simulink model "NeuralcircuitULInjured08102023_DSD"  (R2023a)
settings: Solver=VariableStepAuto  StartTime=0.0  StopTime=1600  RelTol=1e-3
values from neighbouring files (symbols this model uses):
  Cn = 1    [Inhibitory_excitatory_ULInjury_1Hz_08102023.m]    (also in Inhibitory_excitatory_ULInjury_30Hz_08102023.m; InitialExcitatoryInhibitoryNeurons_Healthy08062023.m; InitialExcitatoryInhibitoryULInjured_08102023_DSD.m)
  EK = -84*1    (= -84)    [Inhibitory_excitatory_ULInjury_1Hz_08102023.m]    (also in Inhibitory_excitatory_ULInjury_30Hz_08102023.m; InitialExcitatoryInhibitoryNeurons_Healthy08062023.m; InitialExcitatoryInhibitoryULInjured_08102023_DSD.m)
  EKEx = -90    [Inhibitory_excitatory_ULInjury_1Hz_08102023.m]    (also in Inhibitory_excitatory_ULInjury_30Hz_08102023.m; InitialExcitatoryInhibitoryNeurons_Healthy08062023.m; InitialExcitatoryInhibitoryULInjured_08102023_DSD.m)
  EKIn = -90    [Inhibitory_excitatory_ULInjury_1Hz_08102023.m]    (also in Inhibitory_excitatory_ULInjury_30Hz_08102023.m; InitialExcitatoryInhibitoryNeurons_Healthy08062023.m; InitialExcitatoryInhibitoryULInjured_08102023_DSD.m)
  ELEx = -65    [Inhibitory_excitatory_ULInjury_1Hz_08102023.m]    (also in Inhibitory_excitatory_ULInjury_30Hz_08102023.m; InitialExcitatoryInhibitoryNeurons_Healthy08062023.m; InitialExcitatoryInhibitoryULInjured_08102023_DSD.m)
  ELIn = -65    [Inhibitory_excitatory_ULInjury_1Hz_08102023.m]    (also in Inhibitory_excitatory_ULInjury_30Hz_08102023.m; InitialExcitatoryInhibitoryNeurons_Healthy08062023.m; InitialExcitatoryInhibitoryULInjured_08102023_DSD.m)
  ELk = -83.38*1    (= -83.38)    [Inhibitory_excitatory_ULInjury_1Hz_08102023.m]    (also in Inhibitory_excitatory_ULInjury_30Hz_08102023.m; InitialExcitatoryInhibitoryNeurons_Healthy08062023.m; InitialExcitatoryInhibitoryULInjured_08102023_DSD.m)
  ENa = 50*1    (= 50)    [Inhibitory_excitatory_ULInjury_1Hz_08102023.m]    (also in Inhibitory_excitatory_ULInjury_30Hz_08102023.m; InitialExcitatoryInhibitoryNeurons_Healthy08062023.m; InitialExcitatoryInhibitoryULInjured_08102023_DSD.m)
  ENaEx = 60    [Inhibitory_excitatory_ULInjury_1Hz_08102023.m]    (also in Inhibitory_excitatory_ULInjury_30Hz_08102023.m; InitialExcitatoryInhibitoryNeurons_Healthy08062023.m; InitialExcitatoryInhibitoryULInjured_08102023_DSD.m)
  ENaIn = 55    [Inhibitory_excitatory_ULInjury_1Hz_08102023.m]    (also in Inhibitory_excitatory_ULInjury_30Hz_08102023.m; InitialExcitatoryInhibitoryNeurons_Healthy08062023.m; InitialExcitatoryInhibitoryULInjured_08102023_DSD.m)
  ErestE = -65    [Inhibitory_excitatory_ULInjury_1Hz_08102023.m]    (also in Inhibitory_excitatory_ULInjury_30Hz_08102023.m; InitialExcitatoryInhibitoryNeurons_Healthy08062023.m; InitialExcitatoryInhibitoryULInjured_08102023_DSD.m)
  ErestIn = -64    [Inhibitory_excitatory_ULInjury_1Hz_08102023.m]    (also in Inhibitory_excitatory_ULInjury_30Hz_08102023.m; InitialExcitatoryInhibitoryNeurons_Healthy08062023.m; InitialExcitatoryInhibitoryULInjured_08102023_DSD.m)
  ESynE = -10    [Inhibitory_excitatory_ULInjury_1Hz_08102023.m]    (also in Inhibitory_excitatory_ULInjury_30Hz_08102023.m; InitialExcitatoryInhibitoryNeurons_Healthy08062023.m; InitialExcitatoryInhibitoryULInjured_08102023_DSD.m)
  ESynE2 = -10    [Inhibitory_excitatory_ULInjury_1Hz_08102023.m]    (also in Inhibitory_excitatory_ULInjury_30Hz_08102023.m; InitialExcitatoryInhibitoryNeurons_Healthy08062023.m; InitialExcitatoryInhibitoryULInjured_08102023_DSD.m)
  ESynE3 = -10    [Inhibitory_excitatory_ULInjury_1Hz_08102023.m]    (also in Inhibitory_excitatory_ULInjury_30Hz_08102023.m; InitialExcitatoryInhibitoryNeurons_Healthy08062023.m; InitialExcitatoryInhibitoryULInjured_08102023_DSD.m)
  ESynE4 = -10    [Inhibitory_excitatory_ULInjury_1Hz_08102023.m]    (also in Inhibitory_excitatory_ULInjury_30Hz_08102023.m; InitialExcitatoryInhibitoryNeurons_Healthy08062023.m; InitialExcitatoryInhibitoryULInjured_08102023_DSD.m)
  ESynE5 = -10    [Inhibitory_excitatory_ULInjury_1Hz_08102023.m]    (also in Inhibitory_excitatory_ULInjury_30Hz_08102023.m; InitialExcitatoryInhibitoryNeurons_Healthy08062023.m; InitialExcitatoryInhibitoryULInjured_08102023_DSD.m)
  ESynE6 = -15    [Inhibitory_excitatory_ULInjury_1Hz_08102023.m]    (also in Inhibitory_excitatory_ULInjury_30Hz_08102023.m; InitialExcitatoryInhibitoryNeurons_Healthy08062023.m; InitialExcitatoryInhibitoryULInjured_08102023_DSD.m = -10)
  ESynE7 = -10    [Inhibitory_excitatory_ULInjury_1Hz_08102023.m]    (also in Inhibitory_excitatory_ULInjury_30Hz_08102023.m; InitialExcitatoryInhibitoryNeurons_Healthy08062023.m; InitialExcitatoryInhibitoryULInjured_08102023_DSD.m)
  ESynI = -80    [Inhibitory_excitatory_ULInjury_1Hz_08102023.m]    (also in Inhibitory_excitatory_ULInjury_30Hz_08102023.m; InitialExcitatoryInhibitoryNeurons_Healthy08062023.m; InitialExcitatoryInhibitoryULInjured_08102023_DSD.m)
  ESynI2 = -80    [Inhibitory_excitatory_ULInjury_1Hz_08102023.m]    (also in Inhibitory_excitatory_ULInjury_30Hz_08102023.m; InitialExcitatoryInhibitoryNeurons_Healthy08062023.m; InitialExcitatoryInhibitoryULInjured_08102023_DSD.m)
  ESynI3 = -80    [Inhibitory_excitatory_ULInjury_1Hz_08102023.m]    (also in Inhibitory_excitatory_ULInjury_30Hz_08102023.m; InitialExcitatoryInhibitoryNeurons_Healthy08062023.m; InitialExcitatoryInhibitoryULInjured_08102023_DSD.m)
  ESynI5 = -80    [Inhibitory_excitatory_ULInjury_1Hz_08102023.m]    (also in Inhibitory_excitatory_ULInjury_30Hz_08102023.m; InitialExcitatoryInhibitoryNeurons_Healthy08062023.m; InitialExcitatoryInhibitoryULInjured_08102023_DSD.m)
  ESynI6 = -65    [Inhibitory_excitatory_ULInjury_1Hz_08102023.m]    (also in Inhibitory_excitatory_ULInjury_30Hz_08102023.m; InitialExcitatoryInhibitoryNeurons_Healthy08062023.m; InitialExcitatoryInhibitoryULInjured_08102023_DSD.m = -80)
  Exh0 = ahEx(V0)./(ahEx(V0)+bhEx(V0))    [Inhibitory_excitatory_ULInjury_1Hz_08102023.m]    (also in Inhibitory_excitatory_ULInjury_30Hz_08102023.m; InitialExcitatoryInhibitoryNeurons_Healthy08062023.m; InitialExcitatoryInhibitoryULInjured_08102023_DSD.m)
  Exm0 = amEx(V0)./(amEx(V0)+bmEx(V0))    [Inhibitory_excitatory_ULInjury_1Hz_08102023.m]    (also in Inhibitory_excitatory_ULInjury_30Hz_08102023.m; InitialExcitatoryInhibitoryNeurons_Healthy08062023.m; InitialExcitatoryInhibitoryULInjured_08102023_DSD.m)
  Exn0 = anEx(V0)./(anEx(V0)+bnEx(V0))    [Inhibitory_excitatory_ULInjury_1Hz_08102023.m]    (also in Inhibitory_excitatory_ULInjury_30Hz_08102023.m; InitialExcitatoryInhibitoryNeurons_Healthy08062023.m; InitialExcitatoryInhibitoryULInjured_08102023_DSD.m)
  Ga = 1*Gaxial    (= 0.351233961271)    [Inhibitory_excitatory_ULInjury_1Hz_08102023.m]    (also in Inhibitory_excitatory_ULInjury_30Hz_08102023.m; InitialExcitatoryInhibitoryNeurons_Healthy08062023.m; InitialExcitatoryInhibitoryULInjured_08102023_DSD.m)
  Gaxial = pi*(d^2)/(4*Ro_ax*Internodal_L)*1e7    (= 0.351233961271)    [Inhibitory_excitatory_ULInjury_1Hz_08102023.m]    (also in Inhibitory_excitatory_ULInjury_30Hz_08102023.m; InitialExcitatoryInhibitoryNeurons_Healthy08062023.m; InitialExcitatoryInhibitoryULInjured_08102023_DSD.m)
  gKEx = 100    [Inhibitory_excitatory_ULInjury_1Hz_08102023.m]    (also in Inhibitory_excitatory_ULInjury_30Hz_08102023.m; InitialExcitatoryInhibitoryNeurons_Healthy08062023.m; InitialExcitatoryInhibitoryULInjured_08102023_DSD.m)
  gKIn = 9    [Inhibitory_excitatory_ULInjury_1Hz_08102023.m]    (also in Inhibitory_excitatory_ULInjury_30Hz_08102023.m; InitialExcitatoryInhibitoryNeurons_Healthy08062023.m; InitialExcitatoryInhibitoryULInjured_08102023_DSD.m)
  gKs = 10*0.08/1    (= 0.8)    [Inhibitory_excitatory_ULInjury_1Hz_08102023.m]    (also in Inhibitory_excitatory_ULInjury_30Hz_08102023.m; InitialExcitatoryInhibitoryNeurons_Healthy08062023.m; InitialExcitatoryInhibitoryULInjured_08102023_DSD.m)
  gLEx = 0.1    [Inhibitory_excitatory_ULInjury_1Hz_08102023.m]    (also in Inhibitory_excitatory_ULInjury_30Hz_08102023.m; InitialExcitatoryInhibitoryNeurons_Healthy08062023.m; InitialExcitatoryInhibitoryULInjured_08102023_DSD.m)
  gLIn = 0.1    [Inhibitory_excitatory_ULInjury_1Hz_08102023.m]    (also in Inhibitory_excitatory_ULInjury_30Hz_08102023.m; InitialExcitatoryInhibitoryNeurons_Healthy08062023.m; InitialExcitatoryInhibitoryULInjured_08102023_DSD.m)
  gLk = 10*0.08/1    (= 0.8)    [Inhibitory_excitatory_ULInjury_1Hz_08102023.m]    (also in Inhibitory_excitatory_ULInjury_30Hz_08102023.m; InitialExcitatoryInhibitoryNeurons_Healthy08062023.m; InitialExcitatoryInhibitoryULInjured_08102023_DSD.m)
  gNaEx = 30    [Inhibitory_excitatory_ULInjury_1Hz_08102023.m]    (also in Inhibitory_excitatory_ULInjury_30Hz_08102023.m; InitialExcitatoryInhibitoryNeurons_Healthy08062023.m; InitialExcitatoryInhibitoryULInjured_08102023_DSD.m)
  gNaf = 10*3/1    (= 30)    [Inhibitory_excitatory_ULInjury_1Hz_08102023.m]    (also in Inhibitory_excitatory_ULInjury_30Hz_08102023.m; InitialExcitatoryInhibitoryNeurons_Healthy08062023.m; InitialExcitatoryInhibitoryULInjured_08102023_DSD.m)
  gNaIn = 35    [Inhibitory_excitatory_ULInjury_1Hz_08102023.m]    (also in Inhibitory_excitatory_ULInjury_30Hz_08102023.m; InitialExcitatoryInhibitoryNeurons_Healthy08062023.m; InitialExcitatoryInhibitoryULInjured_08102023_DSD.m)
  gNap = 10*0.005/1    (= 0.05)    [Inhibitory_excitatory_ULInjury_1Hz_08102023.m]    (also in Inhibitory_excitatory_ULInjury_30Hz_08102023.m; InitialExcitatoryInhibitoryNeurons_Healthy08062023.m; InitialExcitatoryInhibitoryULInjured_08102023_DSD.m)
  gSynE = 0.08    [Inhibitory_excitatory_ULInjury_1Hz_08102023.m]    (also in Inhibitory_excitatory_ULInjury_30Hz_08102023.m; InitialExcitatoryInhibitoryNeurons_Healthy08062023.m; InitialExcitatoryInhibitoryULInjured_08102023_DSD.m)
  gSynE2 = 0.08    [Inhibitory_excitatory_ULInjury_1Hz_08102023.m]    (also in Inhibitory_excitatory_ULInjury_30Hz_08102023.m; InitialExcitatoryInhibitoryNeurons_Healthy08062023.m; InitialExcitatoryInhibitoryULInjured_08102023_DSD.m)
  gSynE3 = 0.08    [Inhibitory_excitatory_ULInjury_1Hz_08102023.m]    (also in Inhibitory_excitatory_ULInjury_30Hz_08102023.m; InitialExcitatoryInhibitoryNeurons_Healthy08062023.m; InitialExcitatoryInhibitoryULInjured_08102023_DSD.m)
  gSynE4 = 0.08    [Inhibitory_excitatory_ULInjury_1Hz_08102023.m]    (also in Inhibitory_excitatory_ULInjury_30Hz_08102023.m; InitialExcitatoryInhibitoryNeurons_Healthy08062023.m; InitialExcitatoryInhibitoryULInjured_08102023_DSD.m)
  gSynE5 = 0.08    [Inhibitory_excitatory_ULInjury_1Hz_08102023.m]    (also in Inhibitory_excitatory_ULInjury_30Hz_08102023.m; InitialExcitatoryInhibitoryNeurons_Healthy08062023.m; InitialExcitatoryInhibitoryULInjured_08102023_DSD.m)
  gSynE6 = 0.08    [Inhibitory_excitatory_ULInjury_1Hz_08102023.m]    (also in Inhibitory_excitatory_ULInjury_30Hz_08102023.m; InitialExcitatoryInhibitoryNeurons_Healthy08062023.m; InitialExcitatoryInhibitoryULInjured_08102023_DSD.m)
  gSynE7 = 0.165    [Inhibitory_excitatory_ULInjury_1Hz_08102023.m]    (also in Inhibitory_excitatory_ULInjury_30Hz_08102023.m; InitialExcitatoryInhibitoryNeurons_Healthy08062023.m; InitialExcitatoryInhibitoryULInjured_08102023_DSD.m)
  gSynI = 0.8    [Inhibitory_excitatory_ULInjury_1Hz_08102023.m]    (also in Inhibitory_excitatory_ULInjury_30Hz_08102023.m; InitialExcitatoryInhibitoryNeurons_Healthy08062023.m; InitialExcitatoryInhibitoryULInjured_08102023_DSD.m)
  gSynI2 = 0.12    [Inhibitory_excitatory_ULInjury_1Hz_08102023.m]    (also in Inhibitory_excitatory_ULInjury_30Hz_08102023.m; InitialExcitatoryInhibitoryNeurons_Healthy08062023.m; InitialExcitatoryInhibitoryULInjured_08102023_DSD.m)
  gSynI3 = 0.12    [Inhibitory_excitatory_ULInjury_1Hz_08102023.m]    (also in Inhibitory_excitatory_ULInjury_30Hz_08102023.m; InitialExcitatoryInhibitoryNeurons_Healthy08062023.m; InitialExcitatoryInhibitoryULInjured_08102023_DSD.m)
  gSynI5 = 0.12    [Inhibitory_excitatory_ULInjury_1Hz_08102023.m]    (also in Inhibitory_excitatory_ULInjury_30Hz_08102023.m; InitialExcitatoryInhibitoryNeurons_Healthy08062023.m; InitialExcitatoryInhibitoryULInjured_08102023_DSD.m)
  gSynI6 = 0.12    [Inhibitory_excitatory_ULInjury_1Hz_08102023.m]    (also in Inhibitory_excitatory_ULInjury_30Hz_08102023.m; InitialExcitatoryInhibitoryNeurons_Healthy08062023.m; InitialExcitatoryInhibitoryULInjured_08102023_DSD.m)
  h0 = ah(V0O)./(ah(V0O)+bh(V0O))    [Inhibitory_excitatory_ULInjury_1Hz_08102023.m]    (also in Inhibitory_excitatory_ULInjury_30Hz_08102023.m; InitialExcitatoryInhibitoryNeurons_Healthy08062023.m; InitialExcitatoryInhibitoryULInjured_08102023_DSD.m)
  Inh0 = ahIn(ErestIn)./(ahIn(ErestIn)+bhIn(ErestIn))    [Inhibitory_excitatory_ULInjury_1Hz_08102023.m]    (also in Inhibitory_excitatory_ULInjury_30Hz_08102023.m; InitialExcitatoryInhibitoryNeurons_Healthy08062023.m; InitialExcitatoryInhibitoryULInjured_08102023_DSD.m)
  Inm0 = amIn(ErestIn)./(amIn(ErestIn)+bmIn(ErestIn))    [Inhibitory_excitatory_ULInjury_1Hz_08102023.m]    (also in Inhibitory_excitatory_ULInjury_30Hz_08102023.m; InitialExcitatoryInhibitoryNeurons_Healthy08062023.m; InitialExcitatoryInhibitoryULInjured_08102023_DSD.m)
  Inn0 = anIn(ErestIn)./(anIn(ErestIn)+bnIn(ErestIn))    [Inhibitory_excitatory_ULInjury_1Hz_08102023.m]    (also in Inhibitory_excitatory_ULInjury_30Hz_08102023.m; InitialExcitatoryInhibitoryNeurons_Healthy08062023.m; InitialExcitatoryInhibitoryULInjured_08102023_DSD.m)
  m0 = am(V0O)./(am(V0O)+Bm(V0O))    [Inhibitory_excitatory_ULInjury_1Hz_08102023.m]    (also in Inhibitory_excitatory_ULInjury_30Hz_08102023.m; InitialExcitatoryInhibitoryNeurons_Healthy08062023.m; InitialExcitatoryInhibitoryULInjured_08102023_DSD.m)
  mNap0 = amNap(V0)./(amNap(V0O)+bmNap(V0O))    [Inhibitory_excitatory_ULInjury_1Hz_08102023.m]    (also in Inhibitory_excitatory_ULInjury_30Hz_08102023.m; InitialExcitatoryInhibitoryNeurons_Healthy08062023.m; InitialExcitatoryInhibitoryULInjured_08102023_DSD.m)
  Ro_e = 500    [Inhibitory_excitatory_ULInjury_1Hz_08102023.m]    (also in Inhibitory_excitatory_ULInjury_30Hz_08102023.m; InitialExcitatoryInhibitoryNeurons_Healthy08062023.m; InitialExcitatoryInhibitoryULInjured_08102023_DSD.m)
  s0 = as(V0O)./(as(V0O)+bs(V0O))    [Inhibitory_excitatory_ULInjury_1Hz_08102023.m]    (also in Inhibitory_excitatory_ULInjury_30Hz_08102023.m; InitialExcitatoryInhibitoryNeurons_Healthy08062023.m; InitialExcitatoryInhibitoryULInjured_08102023_DSD.m)
  TawIExt = 30    [Inhibitory_excitatory_ULInjury_1Hz_08102023.m]    (also in Inhibitory_excitatory_ULInjury_30Hz_08102023.m; InitialExcitatoryInhibitoryNeurons_Healthy08062023.m = 200; InitialExcitatoryInhibitoryULInjured_08102023_DSD.m = 200)
  TawIExtE = 30    [Inhibitory_excitatory_ULInjury_1Hz_08102023.m]    (also in Inhibitory_excitatory_ULInjury_30Hz_08102023.m; InitialExcitatoryInhibitoryNeurons_Healthy08062023.m = 1; InitialExcitatoryInhibitoryULInjured_08102023_DSD.m = 10)
  TawSynE = 5    [Inhibitory_excitatory_ULInjury_1Hz_08102023.m]    (also in Inhibitory_excitatory_ULInjury_30Hz_08102023.m; InitialExcitatoryInhibitoryNeurons_Healthy08062023.m; InitialExcitatoryInhibitoryULInjured_08102023_DSD.m)
  TawSynE2 = 11    [Inhibitory_excitatory_ULInjury_1Hz_08102023.m]    (also in Inhibitory_excitatory_ULInjury_30Hz_08102023.m; InitialExcitatoryInhibitoryNeurons_Healthy08062023.m = 12; InitialExcitatoryInhibitoryULInjured_08102023_DSD.m = 5)
  TawSynE3 = 10    [Inhibitory_excitatory_ULInjury_1Hz_08102023.m]    (also in Inhibitory_excitatory_ULInjury_30Hz_08102023.m; InitialExcitatoryInhibitoryNeurons_Healthy08062023.m = 18; InitialExcitatoryInhibitoryULInjured_08102023_DSD.m = 8)
  TawSynE4 = 6    [Inhibitory_excitatory_ULInjury_1Hz_08102023.m]    (also in Inhibitory_excitatory_ULInjury_30Hz_08102023.m; InitialExcitatoryInhibitoryNeurons_Healthy08062023.m; InitialExcitatoryInhibitoryULInjured_08102023_DSD.m)
  TawSynE41 = 14    [Inhibitory_excitatory_ULInjury_1Hz_08102023.m]    (also in Inhibitory_excitatory_ULInjury_30Hz_08102023.m; InitialExcitatoryInhibitoryNeurons_Healthy08062023.m = 15; InitialExcitatoryInhibitoryULInjured_08102023_DSD.m = 6)
  TawSynE5 = 6    [Inhibitory_excitatory_ULInjury_1Hz_08102023.m]    (also in Inhibitory_excitatory_ULInjury_30Hz_08102023.m; InitialExcitatoryInhibitoryNeurons_Healthy08062023.m; InitialExcitatoryInhibitoryULInjured_08102023_DSD.m)
  TawSynE6 = 3    [Inhibitory_excitatory_ULInjury_1Hz_08102023.m]    (also in Inhibitory_excitatory_ULInjury_30Hz_08102023.m; InitialExcitatoryInhibitoryNeurons_Healthy08062023.m; InitialExcitatoryInhibitoryULInjured_08102023_DSD.m)
  TawSynE66 = 1    [Inhibitory_excitatory_ULInjury_1Hz_08102023.m]    (also in Inhibitory_excitatory_ULInjury_30Hz_08102023.m; InitialExcitatoryInhibitoryNeurons_Healthy08062023.m; InitialExcitatoryInhibitoryULInjured_08102023_DSD.m)
  TawSynE66E = 5    [Inhibitory_excitatory_ULInjury_1Hz_08102023.m]    (also in Inhibitory_excitatory_ULInjury_30Hz_08102023.m; InitialExcitatoryInhibitoryNeurons_Healthy08062023.m; InitialExcitatoryInhibitoryULInjured_08102023_DSD.m)
  TawSynE7 = 0.05    [Inhibitory_excitatory_ULInjury_1Hz_08102023.m]    (also in Inhibitory_excitatory_ULInjury_30Hz_08102023.m; InitialExcitatoryInhibitoryNeurons_Healthy08062023.m; InitialExcitatoryInhibitoryULInjured_08102023_DSD.m)
  TawSynI = 5    [Inhibitory_excitatory_ULInjury_1Hz_08102023.m]    (also in Inhibitory_excitatory_ULInjury_30Hz_08102023.m; InitialExcitatoryInhibitoryNeurons_Healthy08062023.m; InitialExcitatoryInhibitoryULInjured_08102023_DSD.m)
  TawSynI2 = 1    [Inhibitory_excitatory_ULInjury_1Hz_08102023.m]    (also in Inhibitory_excitatory_ULInjury_30Hz_08102023.m; InitialExcitatoryInhibitoryNeurons_Healthy08062023.m; InitialExcitatoryInhibitoryULInjured_08102023_DSD.m = 2)
  TawSynI3 = 30    [Inhibitory_excitatory_ULInjury_1Hz_08102023.m]    (also in Inhibitory_excitatory_ULInjury_30Hz_08102023.m; InitialExcitatoryInhibitoryNeurons_Healthy08062023.m = 35; InitialExcitatoryInhibitoryULInjured_08102023_DSD.m)
  TawSynI5 = 4    [Inhibitory_excitatory_ULInjury_1Hz_08102023.m]    (also in Inhibitory_excitatory_ULInjury_30Hz_08102023.m; InitialExcitatoryInhibitoryNeurons_Healthy08062023.m = 1; InitialExcitatoryInhibitoryULInjured_08102023_DSD.m = 1)
  TawSynI6 = 3    [Inhibitory_excitatory_ULInjury_1Hz_08102023.m]    (also in Inhibitory_excitatory_ULInjury_30Hz_08102023.m; InitialExcitatoryInhibitoryNeurons_Healthy08062023.m; InitialExcitatoryInhibitoryULInjured_08102023_DSD.m)
  TawSynI7 = 0.01    [Inhibitory_excitatory_ULInjury_1Hz_08102023.m]    (also in Inhibitory_excitatory_ULInjury_30Hz_08102023.m; InitialExcitatoryInhibitoryNeurons_Healthy08062023.m; InitialExcitatoryInhibitoryULInjured_08102023_DSD.m)
  V0 = -65    [Inhibitory_excitatory_ULInjury_1Hz_08102023.m]    (also in Inhibitory_excitatory_ULInjury_30Hz_08102023.m; InitialExcitatoryInhibitoryNeurons_Healthy08062023.m; InitialExcitatoryInhibitoryULInjured_08102023_DSD.m)
  V0In = -64    [Inhibitory_excitatory_ULInjury_1Hz_08102023.m]    (also in Inhibitory_excitatory_ULInjury_30Hz_08102023.m; InitialExcitatoryInhibitoryNeurons_Healthy08062023.m; InitialExcitatoryInhibitoryULInjured_08102023_DSD.m)
  w12 = -0.2    [Inhibitory_excitatory_ULInjury_1Hz_08102023.m]    (also in Inhibitory_excitatory_ULInjury_30Hz_08102023.m; InitialExcitatoryInhibitoryNeurons_Healthy08062023.m = -0.28; InitialExcitatoryInhibitoryULInjured_08102023_DSD.m = -0.35)
  w14 = 0.05    [Inhibitory_excitatory_ULInjury_1Hz_08102023.m]    (also in Inhibitory_excitatory_ULInjury_30Hz_08102023.m; InitialExcitatoryInhibitoryNeurons_Healthy08062023.m = 0.09; InitialExcitatoryInhibitoryULInjured_08102023_DSD.m = 0.09)
  w15 = -0.45    [Inhibitory_excitatory_ULInjury_1Hz_08102023.m]    (also in Inhibitory_excitatory_ULInjury_30Hz_08102023.m = -0.07; InitialExcitatoryInhibitoryNeurons_Healthy08062023.m = -0.4; InitialExcitatoryInhibitoryULInjured_08102023_DSD.m = -0.4)
  w17 = -0.25    [Inhibitory_excitatory_ULInjury_1Hz_08102023.m]    (also in Inhibitory_excitatory_ULInjury_30Hz_08102023.m; InitialExcitatoryInhibitoryNeurons_Healthy08062023.m; InitialExcitatoryInhibitoryULInjured_08102023_DSD.m)
  w26 = 0.2    [Inhibitory_excitatory_ULInjury_1Hz_08102023.m]    (also in Inhibitory_excitatory_ULInjury_30Hz_08102023.m = 0.25; InitialExcitatoryInhibitoryNeurons_Healthy08062023.m = 0.05; InitialExcitatoryInhibitoryULInjured_08102023_DSD.m = 0.05)
  w28 = 0.165    [Inhibitory_excitatory_ULInjury_1Hz_08102023.m]    (also in Inhibitory_excitatory_ULInjury_30Hz_08102023.m; InitialExcitatoryInhibitoryNeurons_Healthy08062023.m = 0.13; InitialExcitatoryInhibitoryULInjured_08102023_DSD.m = 0.13)
  w34 = 0.09    [Inhibitory_excitatory_ULInjury_1Hz_08102023.m]    (also in Inhibitory_excitatory_ULInjury_30Hz_08102023.m; InitialExcitatoryInhibitoryNeurons_Healthy08062023.m = 0.03; InitialExcitatoryInhibitoryULInjured_08102023_DSD.m = 0.06)
  w63 = -0.12    [Inhibitory_excitatory_ULInjury_1Hz_08102023.m]    (also in Inhibitory_excitatory_ULInjury_30Hz_08102023.m; InitialExcitatoryInhibitoryNeurons_Healthy08062023.m = -0.08; InitialExcitatoryInhibitoryULInjured_08102023_DSD.m = -0.27)
  w66 = 0.03    [Inhibitory_excitatory_ULInjury_1Hz_08102023.m]    (also in Inhibitory_excitatory_ULInjury_30Hz_08102023.m; InitialExcitatoryInhibitoryNeurons_Healthy08062023.m; InitialExcitatoryInhibitoryULInjured_08102023_DSD.m)
  w66E = 0.2    [Inhibitory_excitatory_ULInjury_1Hz_08102023.m]    (also in Inhibitory_excitatory_ULInjury_30Hz_08102023.m; InitialExcitatoryInhibitoryNeurons_Healthy08062023.m = 0.09; InitialExcitatoryInhibitoryULInjured_08102023_DSD.m = 0.1)
  w67 = -0.4    [Inhibitory_excitatory_ULInjury_1Hz_08102023.m]    (also in Inhibitory_excitatory_ULInjury_30Hz_08102023.m; InitialExcitatoryInhibitoryNeurons_Healthy08062023.m = -0.55; InitialExcitatoryInhibitoryULInjured_08102023_DSD.m = -0.55)
  w68 = 0.35    [Inhibitory_excitatory_ULInjury_1Hz_08102023.m]    (also in Inhibitory_excitatory_ULInjury_30Hz_08102023.m; InitialExcitatoryInhibitoryNeurons_Healthy08062023.m = 0.1; InitialExcitatoryInhibitoryULInjured_08102023_DSD.m = 0.1)
  w71 = 0.25    [Inhibitory_excitatory_ULInjury_1Hz_08102023.m]    (also in Inhibitory_excitatory_ULInjury_30Hz_08102023.m; InitialExcitatoryInhibitoryNeurons_Healthy08062023.m; InitialExcitatoryInhibitoryULInjured_08102023_DSD.m)
  w78 = 0.25    [Inhibitory_excitatory_ULInjury_1Hz_08102023.m]    (also in Inhibitory_excitatory_ULInjury_30Hz_08102023.m; InitialExcitatoryInhibitoryNeurons_Healthy08062023.m; InitialExcitatoryInhibitoryULInjured_08102023_DSD.m)
  w79 = 0.35    [Inhibitory_excitatory_ULInjury_1Hz_08102023.m]    (also in Inhibitory_excitatory_ULInjury_30Hz_08102023.m; InitialExcitatoryInhibitoryNeurons_Healthy08062023.m; InitialExcitatoryInhibitoryULInjured_08102023_DSD.m)
  w83 = 0.2    [Inhibitory_excitatory_ULInjury_1Hz_08102023.m]    (also in Inhibitory_excitatory_ULInjury_30Hz_08102023.m; InitialExcitatoryInhibitoryNeurons_Healthy08062023.m = 0.13; InitialExcitatoryInhibitoryULInjured_08102023_DSD.m = 0.08)
  w85 = 0.1    [Inhibitory_excitatory_ULInjury_1Hz_08102023.m]    (also in Inhibitory_excitatory_ULInjury_30Hz_08102023.m = 0.12; InitialExcitatoryInhibitoryNeurons_Healthy08062023.m = 0.04; InitialExcitatoryInhibitoryULInjured_08102023_DSD.m = 0.05)
  X = nan(node,1)    [Inhibitory_excitatory_ULInjury_1Hz_08102023.m]    (also in Inhibitory_excitatory_ULInjury_30Hz_08102023.m; InitialExcitatoryInhibitoryNeurons_Healthy08062023.m; InitialExcitatoryInhibitoryULInjured_08102023_DSD.m)
  X2 = nan(node2,1)    [Inhibitory_excitatory_ULInjury_1Hz_08102023.m]    (also in Inhibitory_excitatory_ULInjury_30Hz_08102023.m; InitialExcitatoryInhibitoryNeurons_Healthy08062023.m; InitialExcitatoryInhibitoryULInjured_08102023_DSD.m)
  Xelec = Xtotal-Nodal_L*9-Internodal_L*9    (= 0.1152)    [Inhibitory_excitatory_ULInjury_1Hz_08102023.m]    (also in Inhibitory_excitatory_ULInjury_30Hz_08102023.m; InitialExcitatoryInhibitoryNeurons_Healthy08062023.m; InitialExcitatoryInhibitoryULInjured_08102023_DSD.m)
  Xelec2 = 1/(10000)+Nodal_L2*(node2-1)/2+Internodal_L2*(node2-1)/2    (= 0.0001)    [Inhibitory_excitatory_ULInjury_1Hz_08102023.m]    (also in Inhibitory_excitatory_ULInjury_30Hz_08102023.m; InitialExcitatoryInhibitoryNeurons_Healthy08062023.m; InitialExcitatoryInhibitoryULInjured_08102023_DSD.m)
  Y = nan(node,1)    [Inhibitory_excitatory_ULInjury_1Hz_08102023.m]    (also in Inhibitory_excitatory_ULInjury_30Hz_08102023.m; InitialExcitatoryInhibitoryNeurons_Healthy08062023.m; InitialExcitatoryInhibitoryULInjured_08102023_DSD.m)
  Y2 = nan(node2,1)    [Inhibitory_excitatory_ULInjury_1Hz_08102023.m]    (also in Inhibitory_excitatory_ULInjury_30Hz_08102023.m; InitialExcitatoryInhibitoryNeurons_Healthy08062023.m; InitialExcitatoryInhibitoryULInjured_08102023_DSD.m)
  Yelec = 100/10000    (= 0.01)    [Inhibitory_excitatory_ULInjury_1Hz_08102023.m]    (also in Inhibitory_excitatory_ULInjury_30Hz_08102023.m; InitialExcitatoryInhibitoryNeurons_Healthy08062023.m; InitialExcitatoryInhibitoryULInjured_08102023_DSD.m)
  Yelec2 = 500/10000    (= 0.05)    [Inhibitory_excitatory_ULInjury_1Hz_08102023.m]    (also in Inhibitory_excitatory_ULInjury_30Hz_08102023.m; InitialExcitatoryInhibitoryNeurons_Healthy08062023.m; InitialExcitatoryInhibitoryULInjured_08102023_DSD.m)
libraries: simulink x1
(part 2 of 14)

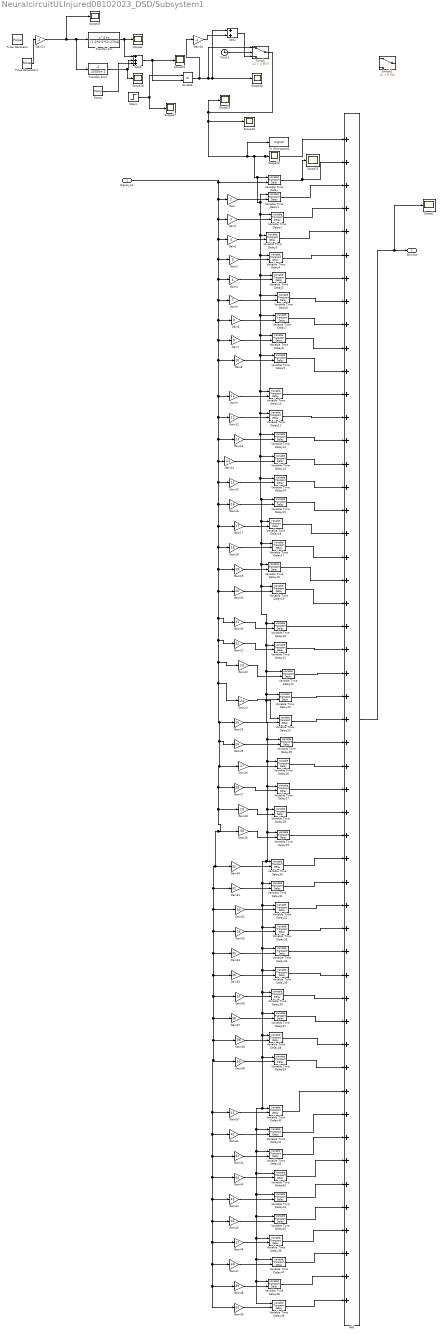
== system NeuralcircuitULInjured08102023_DSD/Subsystem1 ==
  Signal_in1 : Inport
  Add : Sum  Inputs=+++++++++++++++++++++++++++++++++++++++++++++++++++
  Add1 : Sum  Inputs=+++
  Add2 : Sum
  Clock1 : Clock
  Divide3 : Product  Inputs=**
  Gain : Gain  Gain=2
  Gain1 : Gain  Gain=3
  Gain10 : Gain  Gain=-1
  Gain11 : Gain  Gain=-1
  Gain12 : Gain  Gain=12
  Gain13 : Gain  Gain=13
  Gain14 : Gain  Gain=14
  Gain15 : Gain  Gain=15
  Gain16 : Gain  Gain=16
  Gain17 : Gain  Gain=17
  Gain18 : Gain  Gain=18
  Gain19 : Gain  Gain=19
  Gain2 : Gain  Gain=4
  Gain20 : Gain  Gain=20
  Gain21 : Gain  Gain=22
  Gain22 : Gain  Gain=23
  Gain23 : Gain  Gain=24
  Gain24 : Gain  Gain=25
  Gain25 : Gain  Gain=26
  Gain26 : Gain  Gain=27
  Gain27 : Gain  Gain=28
  Gain28 : Gain  Gain=29
  Gain29 : Gain  Gain=30
  Gain3 : Gain  Gain=5
  Gain30 : Gain  Gain=21
  Gain31 : Gain  Gain=32
  Gain32 : Gain  Gain=33
  Gain33 : Gain  Gain=34
  Gain34 : Gain  Gain=35
  Gain35 : Gain  Gain=36
  Gain36 : Gain  Gain=37
  Gain37 : Gain  Gain=38
  Gain38 : Gain  Gain=39
  Gain39 : Gain  Gain=40
  Gain4 : Gain  Gain=6
  Gain40 : Gain  Gain=31
  Gain41 : Gain  Gain=42
  Gain42 : Gain  Gain=43
  Gain43 : Gain  Gain=44
  Gain44 : Gain  Gain=45
  Gain45 : Gain  Gain=46
  Gain46 : Gain  Gain=47
  Gain47 : Gain  Gain=48
  Gain48 : Gain  Gain=49
  Gain49 : Gain  Gain=50
  Gain5 : Gain  Gain=7
  Gain50 : Gain  Gain=41
  Gain6 : Gain  Gain=8
  Gain7 : Gain  Gain=9
  Gain8 : Gain  Gain=10
  Gain9 : Gain  Gain=11
  Pulse Generator : DiscretePulseGenerator  PulseType=Time based  Amplitude=5000  Period=5  PulseWidth=0.5
  Pulse Generator1 : DiscretePulseGenerator  PulseType=Time based  Amplitude=10000  Period=5  PulseWidth=0.05
  Ramp : simulink/Sources/Ramp  slope=0.0002  start=0.05  InitialOutput=0
  Scope{1..2,21..25,27..30} (11 alike) : Scope
  Step1 : Step  Time=2  Before=1  After=0  SampleTime=0
  Switch : Switch  Criteria=u2 > Threshold  Threshold=2.5E-3  SaturateOnIntegerOverflow=off  InputSameDT=off
  Switch1 : Switch  Criteria=u2 > Threshold  Threshold=0.024  SaturateOnIntegerOverflow=off  InputSameDT=off
  To Workspace4 : ToWorkspace  VariableName=signal  SampleTime=-1
  Transfer Fcn : TransferFcn  Numerator=[1 1 0]  Denominator=[1 2*0.5*52 2704]
  Transfer Fcn1 : TransferFcn  Numerator=[-1]  Denominator=[1000 1]
  Variable Time Delay{,1..9,19,29,39,49} (14 alike) : VariableTransportDelay  MaximumDelay=10000
  Variable Time Delay{10..18,20..28,30..38,40..48} (36 alike) : VariableTransportDelay  MaximumDelay=100000
  StimOut : Outport
  wires:
  Gain6/1 -> Variable Time Delay7/2
  Gain4/1 -> Variable Time Delay5/2
  Gain/1 -> Variable Time Delay1/2
  Gain5/1 -> Variable Time Delay6/2
  Gain2/1 -> Variable Time Delay3/2
  Transfer Fcn1/1 -> Scope28/1, Add1/2
  Add2/1 -> Switch/3
  Divide3/1 -> Gain10/1, Switch/1, Scope30/1, Add2/1
  Ramp/1 -> Add1/3
  Gain10/1 -> Add2/2
  Clock1/1 -> Switch/2
  Gain3/1 -> Variable Time Delay4/2
  Gain7/1 -> Variable Time Delay8/2
  Gain11/1 -> Scope29/1, Transfer Fcn1/1, Transfer Fcn/1
  Step1/1 -> Divide3/1, Scope27/1
  Add1/1 -> Divide3/2, Scope21/1
  Transfer Fcn/1 -> Add1/1, Scope1/1
  Variable Time Delay/1 -> Scope23/1, Add/2
  Gain1/1 -> Variable Time Delay2/2
  Gain8/1 -> Variable Time Delay9/2
  Add/1 -> Scope2/1, StimOut/1
  Pulse Generator1/1 -> Gain11/1
  Variable Time Delay1/1 -> Add/3
  Variable Time Delay2/1 -> Add/4
  Variable Time Delay3/1 -> Add/5
  Variable Time Delay4/1 -> Add/6
  Variable Time Delay5/1 -> Add/7
  Variable Time Delay6/1 -> Add/8
  Variable Time Delay7/1 -> Add/9
  Variable Time Delay8/1 -> Add/10
  Variable Time Delay9/1 -> Add/11
  Gain9/1 -> Variable Time Delay10/2
  Variable Time Delay10/1 -> Add/12
  Gain12/1 -> Variable Time Delay11/2
  Variable Time Delay11/1 -> Add/13
  Gain13/1 -> Variable Time Delay12/2
  Variable Time Delay12/1 -> Add/14
  Gain14/1 -> Variable Time Delay13/2
  Variable Time Delay13/1 -> Add/15
  Gain15/1 -> Variable Time Delay14/2
  Variable Time Delay14/1 -> Add/16
  Gain16/1 -> Variable Time Delay15/2
  Variable Time Delay15/1 -> Add/17
  Gain17/1 -> Variable Time Delay16/2
  Variable Time Delay16/1 -> Add/18
  Gain18/1 -> Variable Time Delay17/2
  Variable Time Delay17/1 -> Add/19
  Gain19/1 -> Variable Time Delay18/2
  Variable Time Delay18/1 -> Add/20
  Gain20/1 -> Variable Time Delay19/2
  Variable Time Delay19/1 -> Add/21
  Gain21/1 -> Variable Time Delay21/2
  Gain23/1 -> Variable Time Delay23/2
  Gain28/1 -> Variable Time Delay28/2
  Gain30/1 -> Variable Time Delay20/2
  Gain24/1 -> Variable Time Delay24/2
  Gain29/1 -> Variable Time Delay29/2
  Gain26/1 -> Variable Time Delay26/2
  Gain22/1 -> Variable Time Delay22/2
  Gain25/1 -> Variable Time Delay25/2
  Gain27/1 -> Variable Time Delay27/2
  Variable Time Delay20/1 -> Add/22
  Variable Time Delay21/1 -> Add/23
  Variable Time Delay22/1 -> Add/24
  Variable Time Delay23/1 -> Add/25
  Variable Time Delay24/1 -> Add/26
  Variable Time Delay25/1 -> Add/27
  Variable Time Delay26/1 -> Add/28
  Variable Time Delay27/1 -> Add/29
  Variable Time Delay28/1 -> Add/30
  Variable Time Delay29/1 -> Add/31
  Variable Time Delay30/1 -> Add/32
  Variable Time Delay36/1 -> Add/38
  Gain33/1 -> Variable Time Delay33/2
  Variable Time Delay31/1 -> Add/33
  Gain31/1 -> Variable Time Delay31/2
  Gain40/1 -> Variable Time Delay30/2
  Gain38/1 -> Variable Time Delay38/2
  Gain37/1 -> Variable Time Delay37/2
  Variable Time Delay38/1 -> Add/40
  Gain35/1 -> Variable Time Delay35/2
  Gain39/1 -> Variable Time Delay39/2
  Gain36/1 -> Variable Time Delay36/2
  Gain34/1 -> Variable Time Delay34/2
  Gain32/1 -> Variable Time Delay32/2
  Variable Time Delay32/1 -> Add/34
  Variable Time Delay33/1 -> Add/35
  Variable Time Delay34/1 -> Add/36
  Variable Time Delay35/1 -> Add/37
  Variable Time Delay37/1 -> Add/39
  Variable Time Delay39/1 -> Add/41
  Switch/1 -> Scope25/1, Scope22/1, To Workspace4/1, Variable Time Delay3/1, Variable Time Delay4/1, Variable Time Delay6/1, Variable Time Delay8/1, Variable Time Delay49/1, Variable Time Delay48/1, Variable Time Delay47/1, Variable Time Delay46/1, Variable Time Delay45/1, Variable Time Delay44/1, Variable Time Delay43/1, Variable Time Delay42/1, Variable Time Delay41/1, Variable Time Delay40/1, Variable Time Delay39/1, Variable Time Delay38/1, Variable Time Delay37/1, Variable Time Delay36/1, Variable Time Delay35/1, Variable Time Delay34/1, Variable Time Delay33/1, Variable Time Delay32/1, Variable Time Delay31/1, Variable Time Delay30/1, Variable Time Delay29/1, Variable Time Delay28/1, Variable Time Delay27/1, Variable Time Delay26/1, Variable Time Delay25/1, Variable Time Delay24/1, Variable Time Delay23/1, Variable Time Delay22/1, Variable Time Delay21/1, Variable Time Delay20/1, Variable Time Delay19/1, Variable Time Delay18/1, Variable Time Delay17/1, Variable Time Delay16/1, Variable Time Delay15/1, Variable Time Delay14/1, Variable Time Delay13/1, Variable Time Delay12/1, Variable Time Delay11/1, Variable Time Delay10/1, Variable Time Delay9/1, Variable Time Delay7/1, Variable Time Delay5/1, Variable Time Delay2/1, Variable Time Delay1/1, Variable Time Delay/1, Add/1, Scope24/1
  Gain48/1 -> Variable Time Delay48/2
  Gain44/1 -> Variable Time Delay44/2
  Gain46/1 -> Variable Time Delay46/2
  Gain45/1 -> Variable Time Delay45/2
  Gain49/1 -> Variable Time Delay49/2
  Gain41/1 -> Variable Time Delay41/2
  Gain43/1 -> Variable Time Delay43/2
  Signal_in1/1 -> Gain8/1, Gain14/1, Gain16/1, Gain17/1, Gain18/1, Gain19/1, Gain30/1, Gain21/1, Gain22/1, Gain23/1, Gain24/1, Gain25/1, Gain29/1, Gain40/1, Gain31/1, Gain32/1, Gain33/1, Gain34/1, Gain35/1, Gain36/1, Gain37/1, Gain38/1, Gain50/1, Gain41/1, Gain42/1, Gain43/1, Gain44/1, Gain45/1, Gain46/1, Gain47/1, Gain48/1, Gain49/1, Gain39/1, Gain28/1, Gain27/1, Gain26/1, Gain20/1, Gain15/1, Gain13/1, Gain12/1, Gain9/1, Gain7/1, Gain6/1, Gain5/1, Gain4/1, Gain3/1, Gain2/1, Gain1/1, Gain/1, Variable Time Delay/2
  Gain47/1 -> Variable Time Delay47/2
  Gain50/1 -> Variable Time Delay40/2
  Gain42/1 -> Variable Time Delay42/2
  Variable Time Delay40/1 -> Add/42
  Variable Time Delay41/1 -> Add/43
  Variable Time Delay42/1 -> Add/44
  Variable Time Delay43/1 -> Add/45
  Variable Time Delay44/1 -> Add/46
  Variable Time Delay45/1 -> Add/47
  Variable Time Delay46/1 -> Add/48
  Variable Time Delay47/1 -> Add/49
  Variable Time Delay48/1 -> Add/50
  Variable Time Delay49/1 -> Add/51

== system NeuralcircuitULInjured08102023_DSD/excitatory Neuron 1 ==
  Iext : Inport
  Xj : Inport  Port=2
  Yj : Inport  Port=3
  "I " : Inport  Port=4
  VPreE7 : Inport  Port=5
  Add : Sum  Inputs=+---++-
  Add1 : Sum  Inputs=+-
  Constant2 : Constant  Value=ENaEx
  Divide : Product  Inputs=**
  Gain : Gain  Gain=1/Cn
  Integrator : Integrator  InitialCondition=V0
  Ks : Subsystem
  Lk : Subsystem
  Naf : Subsystem
  Nap1 : Subsystem
  Scope{1..3,5} (4 alike) : Scope
  Selector : Selector  InputPortWidth=1  IndexOptions=Index vector (dialog)  Indices=p  OutputSizes=1
  Selector1 : Selector  InputPortWidth=1  IndexOptions=Index vector (dialog)  Indices=p  OutputSizes=1
  Subsystem : Subsystem
  Transfer Fcn1 : TransferFcn  Denominator=[TawIExt 1]
  Vm : Outport  VectorParamsAs1DForOutWhenUnconnected=off
  wires:
  Divide/1 -> Add/1
  Ks/1(IKs) -> Add/3
  Naf/1("INaf ") -> Add/2
  Add/1 -> Scope3/1, Gain/1
  Lk/1(ILk) -> Scope5/1, Add/4
  Transfer Fcn1/1 -> Divide/2, Scope1/1
  Gain/1 -> Integrator/1
  Subsystem/1(ku) -> Transfer Fcn1/1
  Xj/1 -> Selector/1
  Iext/1 -> Subsystem/1(Iext)
  Selector/1 -> Subsystem/2(Xj)
  Selector1/1 -> Subsystem/3(Yj)
  Yj/1 -> Selector1/1
  "I "/1 -> Add/5
  Add1/1 -> Divide/1
  Constant2/1 -> Add1/1
  Integrator/1 -> Naf/1(Vm), Add1/2, Ks/1(Vm), Lk/1(Vm), Nap1/1(V), Vm/1
  Nap1/1("ISynE ") -> Add/7
  VPreE7/1 -> Nap1/2(Pre)

== system NeuralcircuitULInjured08102023_DSD/excitatory Neuron 1-1 ==
  Iext : Inport
  Xj : Inport  Port=2
  Yj : Inport  Port=3
  "I " : Inport  Port=4
  VPreE1 : Inport  Port=5
  Add : Sum  Inputs=+---++-
  Add1 : Sum  Inputs=+-
  Constant2 : Constant  Value=ENaEx
  Divide : Product  Inputs=**
  Gain : Gain  Gain=1/Cn
  Integrator : Integrator  InitialCondition=V0
  Ks : Subsystem
  Lk : Subsystem
  Naf : Subsystem
  Nap1 : Subsystem
  Scope{1..3,5} (4 alike) : Scope
  Selector : Selector  InputPortWidth=1  IndexOptions=Index vector (dialog)  Indices=p  OutputSizes=1
  Selector1 : Selector  InputPortWidth=1  IndexOptions=Index vector (dialog)  Indices=p  OutputSizes=1
  Subsystem : Subsystem
  Transfer Fcn1 : TransferFcn  Denominator="[TawIExtE  1]"
  Vm : Outport  VectorParamsAs1DForOutWhenUnconnected=off
  wires:
  Divide/1 -> Add/1
  Ks/1(IKs) -> Add/3
  Naf/1("INaf ") -> Add/2
  Add/1 -> Scope3/1, Gain/1
  Lk/1(ILk) -> Scope5/1, Add/4
  Transfer Fcn1/1 -> Divide/2, Scope1/1
  Gain/1 -> Integrator/1
  Subsystem/1(ku) -> Transfer Fcn1/1
  Xj/1 -> Selector/1
  Iext/1 -> Subsystem/1(Iext)
  Selector/1 -> Subsystem/2(Xj)
  Selector1/1 -> Subsystem/3(Yj)
  Yj/1 -> Selector1/1
  "I "/1 -> Add/5
  Add1/1 -> Divide/1
  Constant2/1 -> Add1/1
  Integrator/1 -> Naf/1(Vm), Add1/2, Ks/1(Vm), Lk/1(Vm), Nap1/1(V), Vm/1
  Nap1/1("ISynE ") -> Add/7
  VPreE1/1 -> Nap1/2(Pre)

== system NeuralcircuitULInjured08102023_DSD/excitatory Neuron 2 ==
  Iext : Inport
  Xj : Inport  Port=2
  Yj : Inport  Port=3
  "I " : Inport  Port=4
  "VPre1I " : Inport  Port=5
  VPre6E : Inport  Port=6
  VPre1I : Inport  Port=7
  VPre8E : Inport  Port=8
  Add : Sum  Inputs=+---++----
  Add1 : Sum  Inputs=+-
  Constant2 : Constant  Value=ENaEx
  Divide : Product  Inputs=**
  Gain : Gain  Gain=1/Cn
  Integrator : Integrator  InitialCondition=V0
  Ks : Subsystem
  Lk : Subsystem
  Naf : Subsystem
  Nap1 : Subsystem
  Nap2 : Subsystem
  Nap3 : Subsystem
  Nap4 : Subsystem
  Scope{1..3,5} (4 alike) : Scope
  Selector : Selector  InputPortWidth=1  IndexOptions=Index vector (dialog)  Indices=p  OutputSizes=1
  Selector1 : Selector  InputPortWidth=1  IndexOptions=Index vector (dialog)  Indices=p  OutputSizes=1
  Subsystem : Subsystem
  Transfer Fcn1 : TransferFcn  Denominator=[TawIExtE 1]
  Vm : Outport  VectorParamsAs1DForOutWhenUnconnected=off
  wires:
  Divide/1 -> Add/1
  Ks/1(IKs) -> Add/3
  Naf/1("INaf ") -> Add/2
  Add/1 -> Scope3/1, Gain/1
  Lk/1(ILk) -> Add/4, Scope5/1
  Transfer Fcn1/1 -> Divide/2, Scope1/1
  Gain/1 -> Integrator/1
  Subsystem/1(ku) -> Transfer Fcn1/1
  Xj/1 -> Selector/1
  Iext/1 -> Subsystem/1(Iext)
  Selector/1 -> Subsystem/2(Xj)
  Selector1/1 -> Subsystem/3(Yj)
  Yj/1 -> Selector1/1
  "I "/1 -> Add/5
  Add1/1 -> Divide/1
  Constant2/1 -> Add1/1
  Integrator/1 -> Nap4/1(V), Nap1/1(V), Add1/2, Naf/1(Vm), Ks/1(Vm), Lk/1(Vm), Nap2/1(V), Nap3/1(V), Vm/1
  Nap2/1("ISynI ") -> Add/8
  Nap1/1("ISynE ") -> Scope2/1, Add/7
  VPre8E/1 -> Nap4/2(Pre2)
  VPre1I/1 -> Nap3/2(Pre)
  Nap3/1("ISynI ") -> Add/9
  Nap4/1("ISynE ") -> Add/10
  VPre6E/1 -> Nap1/2(Pre2)

== system NeuralcircuitULInjured08102023_DSD/excitatory Neuron 3 ==
  Iext : Inport
  Xj : Inport  Port=2
  Yj : Inport  Port=3
  "I " : Inport  Port=4
  "VPreI " : Inport  Port=5
  VPre8E : Inport  Port=6
  Add : Sum  Inputs=+---++--
  Add1 : Sum  Inputs=+-
  Constant2 : Constant  Value=ENaEx
  Divide : Product  Inputs=**
  Gain : Gain  Gain=1/Cn
  Integrator : Integrator  InitialCondition=V0
  Ks : Subsystem
  Lk : Subsystem
  Naf : Subsystem
  Nap4 : Subsystem
  Nap5 : Subsystem
  Scope{1..8} (8 alike) : Scope
  Selector : Selector  InputPortWidth=1  IndexOptions=Index vector (dialog)  Indices=p  OutputSizes=1
  Selector1 : Selector  InputPortWidth=1  IndexOptions=Index vector (dialog)  Indices=p  OutputSizes=1
  Subsystem : Subsystem
  Transfer Fcn1 : TransferFcn  Denominator=[TawIExt 1]
  Vm : Outport  VectorParamsAs1DForOutWhenUnconnected=off
  wires:
  Divide/1 -> Add/1
  Ks/1(IKs) -> Scope4/1, Add/3
  Naf/1("INaf ") -> Scope6/1, Add/2
  Add/1 -> Scope3/1, Gain/1
  Lk/1(ILk) -> Add/4, Scope5/1
  Transfer Fcn1/1 -> Divide/2, Scope1/1
  Gain/1 -> Integrator/1
  Subsystem/1(ku) -> Transfer Fcn1/1
  Xj/1 -> Selector/1
  Iext/1 -> Subsystem/1(Iext)
  Selector/1 -> Subsystem/2(Xj)
  Selector1/1 -> Subsystem/3(Yj)
  Yj/1 -> Selector1/1
  "I "/1 -> Add/5
  Add1/1 -> Divide/1
  Constant2/1 -> Add1/1
  VPre8E/1 -> Nap5/2(Pre)
  Integrator/1 -> Scope2/1, Nap4/1(V), Lk/1(Vm), Ks/1(Vm), Naf/1(Vm), Add1/2, Nap5/1(V), Vm/1
  "VPreI "/1 -> Nap4/2(Pre)
  Nap4/1("ISynI ") -> Scope8/1, Add/7
  Nap5/1("ISynE ") -> Scope7/1, Add/8

== system NeuralcircuitULInjured08102023_DSD/excitatory Neuron 4 ==
  Iext : Inport
  Xj : Inport  Port=2
  Yj : Inport  Port=3
  "I " : Inport  Port=4
  "VPre1E " : Inport  Port=5
  VPre3E : Inport  Port=6
  Add : Sum  Inputs=+---++----
  Add1 : Sum  Inputs=+-
  Constant2 : Constant  Value=ENaEx
  Divide : Product  Inputs=**
  Gain : Gain  Gain=1/Cn
  Integrator : Integrator  InitialCondition=-65
  Ks : Subsystem
  Lk : Subsystem
  Naf : Subsystem
  Nap1 : Subsystem
  Nap3 : Subsystem
  Scope{1..5} (5 alike) : Scope
  Selector : Selector  InputPortWidth=1  IndexOptions=Index vector (dialog)  Indices=p  OutputSizes=1
  Selector1 : Selector  InputPortWidth=1  IndexOptions=Index vector (dialog)  Indices=p  OutputSizes=1
  Subsystem : Subsystem
  Transfer Fcn1 : TransferFcn  Denominator=[TawIExt 1]
  Vm : Outport  VectorParamsAs1DForOutWhenUnconnected=off
  wires:
  Divide/1 -> Add/1
  Ks/1(IKs) -> Add/3
  Naf/1("INaf ") -> Add/2
  Add/1 -> Scope3/1, Gain/1
  Lk/1(ILk) -> Add/4, Scope5/1
  Transfer Fcn1/1 -> Divide/2, Scope1/1
  Gain/1 -> Integrator/1
  Subsystem/1(ku) -> Transfer Fcn1/1
  Xj/1 -> Selector/1
  Iext/1 -> Subsystem/1(Iext)
  Selector/1 -> Subsystem/2(Xj)
  Selector1/1 -> Subsystem/3(Yj)
  Yj/1 -> Selector1/1
  "I "/1 -> Add/5
  Add1/1 -> Divide/1
  Constant2/1 -> Add1/1
  VPre3E/1 -> Nap3/2(Pre)
  Nap1/1("ISynE ") -> Add/7
  Nap3/1("ISynE ") -> Scope4/1, Add/9
  Integrator/1 -> Scope2/1, Nap3/1(V), Add1/2, Naf/1(Vm), Ks/1(Vm), Lk/1(Vm), Nap1/1(V), Vm/1
  "VPre1E "/1 -> Nap1/2(Pre)

== system NeuralcircuitULInjured08102023_DSD/excitatory Neuron 6_1 ==
  Iext : Inport
  Xj : Inport  Port=2
  Yj : Inport  Port=3
  "I " : Inport  Port=4
  VPre6E : Inport  Port=5
  Add : Sum  Inputs=+---++--
  Add1 : Sum  Inputs=+-
  Constant2 : Constant  Value=ENaEx
  Divide : Product  Inputs=**
  Gain : Gain  Gain=1/Cn
  Integrator : Integrator  InitialCondition=V0
  Ks : Subsystem
  Lk : Subsystem
  Naf : Subsystem
  Nap1 : Subsystem
  Scope{1..7} (7 alike) : Scope
  Selector : Selector  InputPortWidth=1  IndexOptions=Index vector (dialog)  Indices=p  OutputSizes=1
  Selector1 : Selector  InputPortWidth=1  IndexOptions=Index vector (dialog)  Indices=p  OutputSizes=1
  Subsystem : Subsystem
  Transfer Fcn1 : TransferFcn  Denominator="[TawIExtE  1]"
  Vm : Outport  VectorParamsAs1DForOutWhenUnconnected=off
  wires:
  Divide/1 -> Add/1
  Ks/1(IKs) -> Scope6/1, Add/3
  Naf/1("INaf ") -> Scope7/1, Add/2
  Add/1 -> Scope3/1, Gain/1
  Lk/1(ILk) -> Add/4, Scope5/1
  Transfer Fcn1/1 -> Divide/2, Scope1/1
  Gain/1 -> Integrator/1
  Subsystem/1(ku) -> Scope4/1, Transfer Fcn1/1
  Xj/1 -> Selector/1
  Iext/1 -> Subsystem/1(Iext)
  Selector/1 -> Subsystem/2(Xj)
  Selector1/1 -> Subsystem/3(Yj)
  Yj/1 -> Selector1/1
  "I "/1 -> Add/5
  Add1/1 -> Divide/1
  Constant2/1 -> Add1/1
  Integrator/1 -> Scope2/1, Vm/1, Nap1/1(V), Add1/2, Naf/1(Vm), Ks/1(Vm), Lk/1(Vm)
  ? -> Add/8
  Nap1/1("ISynE ") -> Add/7
  VPre6E/1 -> Nap1/2(Pre)

== system NeuralcircuitULInjured08102023_DSD/Inhibitory Neuron 1/Ks ==
  Vm : Inport
  Add : Sum  Inputs=-+
  Constant : Constant  Value=gKIn
  Constant1 : Constant  Value=EKIn
  Divide : Product  Inputs=*****
  Divide1 : Product  Inputs=**
  "n " : Subsystem
  IKs : Outport  VectorParamsAs1DForOutWhenUnconnected=off
  wires:
  Constant1/1 -> Add/1
  Add/1 -> Divide1/2
  Divide1/1 -> IKs/1
  Divide/1 -> Divide1/1
  [Vm] -> "n "/1(Vm)
  Vm/1 -> Add/2, [Vm]
  Constant/1 -> Divide/5
  "n "/1(n) -> Divide/3, Divide/4, Divide/2, Divide/1

== system NeuralcircuitULInjured08102023_DSD/Inhibitory Neuron 1/Lk ==
  Vm : Inport
  Add : Sum  Inputs=-+
  Constant : Constant  Value=gLIn
  Constant1 : Constant  Value=ELIn
  Divide1 : Product  Inputs=**
  ILk : Outport  VectorParamsAs1DForOutWhenUnconnected=off
  wires:
  Constant1/1 -> Add/1
  Add/1 -> Divide1/2
  Divide1/1 -> ILk/1
  Vm/1 -> Add/2, [Vm]
  Constant/1 -> Divide1/1

== system NeuralcircuitULInjured08102023_DSD/Inhibitory Neuron 1/Naf ==
  Vm : Inport
  Add : Sum  Inputs=-+
  Constant : Constant  Value=gNaIn
  Constant1 : Constant  Value=ENaIn
  Divide : Product  Inputs=*****
  Divide1 : Product  Inputs=**
  h : Subsystem
  "m " : Subsystem
  "INaf " : Outport  VectorParamsAs1DForOutWhenUnconnected=off
  wires:
  Constant1/1 -> Add/1
  Constant/1 -> Divide/5
  Add/1 -> Divide1/2
  [Vm] -> h/1(Vi)
  Divide1/1 -> "INaf "/1
  "m "/1(mNaf) -> Divide/3, Divide/2, Divide/1
  h/1(hNaf) -> Divide/4
  Divide/1 -> Divide1/1
  [Vm] -> "m "/1(Vm)
  Vm/1 -> Add/2, [Vm]

== system NeuralcircuitULInjured08102023_DSD/Inhibitory Neuron 1/Nap1 ==
  V : Inport
  Pre : Inport  Port=2
  Add : Sum  Inputs=-+
  Add1 : Sum  Inputs=+-
  Constant : Constant  Value=gSynE
  Constant1 : Constant  Value=ESynE
  Constant3 : Constant  Value=w71
  Constant4 : Constant  Value=-82
  Divide : Product  Inputs=**
  Divide1 : Product  Inputs=***
  Saturation : Saturate  UpperLimit=inf  LowerLimit=0
  Transfer Fcn : TransferFcn  Denominator=[TawSynE 1]
  "ISynE " : Outport  VectorParamsAs1DForOutWhenUnconnected=off
  wires:
  Constant1/1 -> Add/1
  Add/1 -> Divide1/2
  Divide1/1 -> "ISynE "/1
  Constant/1 -> Divide1/1
  V/1 -> Add/2
  Constant3/1 -> Saturation/1
  Saturation/1 -> Divide/1
  Divide/1 -> Divide1/3
  Transfer Fcn/1 -> Divide/2
  Constant4/1 -> Add1/2
  Pre/1 -> Add1/1
  Add1/1 -> Transfer Fcn/1

== system NeuralcircuitULInjured08102023_DSD/Inhibitory Neuron 1/Subsystem ==
  Iext : Inport
  Xj : Inport  Port=2
  Yj : Inport  Port=3
  Add1 : Sum  Inputs=+-
  Add2 : Sum  Inputs=+-
  Add3 : Sum
  Add4 : Sum  Inputs=+-
  Constant1 : Constant  Value=1/30
  Constant2 : Constant  Value=40
  Constant3 : Constant  Value=4
  Constant4 : Constant  Value=pi
  Constant5 : Constant  Value=Xelec2
  Constant6 : Constant  Value=Yelec2
  Constant7 : Constant  Value=0
  Divide{2..6} (5 alike) : Product  Inputs=**
  MinMax : MinMax  Function=max  Inputs=2
  Sqrt : Sqrt
  ku : Outport  VectorParamsAs1DForOutWhenUnconnected=off
  wires:
  Divide5/1 -> Add3/2
  Sqrt/1 -> Divide6/2
  Add2/1 -> Divide5/2, Divide5/1
  Add1/1 -> Divide4/2, Divide4/1
  Xj/1 -> Add1/2
  Add3/1 -> Sqrt/1
  Divide3/1 -> Divide6/1
  Constant3/1 -> Divide3/1
  Constant4/1 -> Divide3/2
  Divide2/1 -> ku/1
  Divide4/1 -> Add3/1
  Yj/1 -> Add2/2
  Constant6/1 -> Add2/1
  Constant5/1 -> Add1/1
  Constant1/1 -> Divide2/2
  Iext/1 -> Divide2/1, Add4/1
  Constant7/1 -> MinMax/2
  Add4/1 -> MinMax/1

== system NeuralcircuitULInjured08102023_DSD/Inhibitory Neuron 1-1/Ks ==
  Vm : Inport
  Add : Sum  Inputs=-+
  Constant : Constant  Value=gKIn
  Constant1 : Constant  Value=EKIn
  Divide : Product  Inputs=*****
  Divide1 : Product  Inputs=**
  "n " : Subsystem
  IKs : Outport  VectorParamsAs1DForOutWhenUnconnected=off
  wires:
  Constant1/1 -> Add/1
  Add/1 -> Divide1/2
  Divide1/1 -> IKs/1
  Divide/1 -> Divide1/1
  [Vm] -> "n "/1(Vm)
  Vm/1 -> Add/2, [Vm]
  Constant/1 -> Divide/5
  "n "/1(n) -> Divide/3, Divide/4, Divide/2, Divide/1

== system NeuralcircuitULInjured08102023_DSD/Inhibitory Neuron 1-1/Lk ==
  Vm : Inport
  Add : Sum  Inputs=-+
  Constant : Constant  Value=gLIn
  Constant1 : Constant  Value=ELIn
  Divide1 : Product  Inputs=**
  ILk : Outport  VectorParamsAs1DForOutWhenUnconnected=off
  wires:
  Constant1/1 -> Add/1
  Add/1 -> Divide1/2
  Divide1/1 -> ILk/1
  Vm/1 -> Add/2, [Vm]
  Constant/1 -> Divide1/1

== system NeuralcircuitULInjured08102023_DSD/Inhibitory Neuron 1-1/Naf ==
  Vm : Inport
  Add : Sum  Inputs=-+
  Constant : Constant  Value=gNaIn
  Constant1 : Constant  Value=ENaIn
  Divide : Product  Inputs=*****
  Divide1 : Product  Inputs=**
  h : Subsystem
  "m " : Subsystem
  "INaf " : Outport  VectorParamsAs1DForOutWhenUnconnected=off
  wires:
  Constant1/1 -> Add/1
  Constant/1 -> Divide/5
  Add/1 -> Divide1/2
  [Vm] -> h/1(Vi)
  Divide1/1 -> "INaf "/1
  "m "/1(mNaf) -> Divide/3, Divide/2, Divide/1
  h/1(hNaf) -> Divide/4
  Divide/1 -> Divide1/1
  [Vm] -> "m "/1(Vm)
  Vm/1 -> Add/2, [Vm]

== system NeuralcircuitULInjured08102023_DSD/Inhibitory Neuron 1-1/Nap1 ==
  V : Inport
  Pre : Inport  Port=2
  Add : Sum  Inputs=-+
  Add1 : Sum  Inputs=+-
  Constant : Constant  Value=gSynE
  Constant1 : Constant  Value=ESynE
  Constant3 : Constant  Value=w71
  Constant4 : Constant  Value=ErestE
  Divide : Product  Inputs=**
  Divide1 : Product  Inputs=***
  Saturation : Saturate  UpperLimit=inf  LowerLimit=0
  Transfer Fcn : TransferFcn  Denominator=[TawSynE 1]
  "ISynE " : Outport  VectorParamsAs1DForOutWhenUnconnected=off
  wires:
  Constant1/1 -> Add/1
  Add/1 -> Divide1/2
  Divide1/1 -> "ISynE "/1
  Constant/1 -> Divide1/1
  V/1 -> Add/2
  Constant3/1 -> Saturation/1
  Saturation/1 -> Divide/1
  Divide/1 -> Divide1/3
  Transfer Fcn/1 -> Divide/2
  Pre/1 -> Add1/1
  Add1/1 -> Transfer Fcn/1

== system NeuralcircuitULInjured08102023_DSD/Inhibitory Neuron 1-1/Subsystem ==
  Iext : Inport
  Xj : Inport  Port=2
  Yj : Inport  Port=3
  Add1 : Sum  Inputs=+-
  Add2 : Sum  Inputs=+-
  Add3 : Sum
  Add4 : Sum  Inputs=+-
  Constant1 : Constant  Value=1/30
  Constant2 : Constant  Value=40
  Constant3 : Constant  Value=4
  Constant4 : Constant  Value=pi
  Constant5 : Constant  Value=Xelec2
  Constant6 : Constant  Value=Yelec2
  Constant7 : Constant  Value=0
  Divide{2..6} (5 alike) : Product  Inputs=**
  MinMax : MinMax  Function=max  Inputs=2
  Sqrt : Sqrt
  ku : Outport  VectorParamsAs1DForOutWhenUnconnected=off
  wires:
  Divide5/1 -> Add3/2
  Sqrt/1 -> Divide6/2
  Add2/1 -> Divide5/2, Divide5/1
  Add1/1 -> Divide4/2, Divide4/1
  Xj/1 -> Add1/2
  Add3/1 -> Sqrt/1
  Divide3/1 -> Divide6/1
  Constant3/1 -> Divide3/1
  Constant4/1 -> Divide3/2
  Divide2/1 -> ku/1
  Divide4/1 -> Add3/1
  Yj/1 -> Add2/2
  Constant6/1 -> Add2/1
  Constant5/1 -> Add1/1
  Constant1/1 -> Divide2/2
  Iext/1 -> Divide2/1, Add4/1
  Constant7/1 -> MinMax/2
  Add4/1 -> MinMax/1
